simulink model "BESS1_pu"  (R2020b)
settings: Solver=ode1  StartTime=0.0  StopTime=160  FixedStep=Ts  RelTol=1e-3
PostLoadFcn:
  | clc; clear all; close all;
  | 
  | % Modulo 10 - Controle Grid-Forming %
  | 
  | vs_ref = 400;
  | Vnom_rms = vs_ref;
  | Vnom_peak = sqrt(2/3)*Vnom_rms;
  | Pnom =29.75e3;
  | Sbase = Pnom;
  | Vdc = 1400;
  | wnom = 2*pi*60;
  | ron = 0.00088;
  | Ron = ron;
  | %%%% To pu %%%%
  | Vbase = Vnom_rms*sqrt(2);
  | V_LG = Vnom_rms/sqrt(3);
  | Ibase = (Pnom*sqrt(2))/(V_LG*3);
  | 
  | Irms = Pnom/(sqrt(3)*Vnom_rms);                     % Ig rms
  | Inom_peak = Irms*sqrt(2);                           % Ig pico
  | Zbase = Vnom_peak/Inom_peak;                        % Impedancia Base
  | Kconv = Zbase;                                      % Ganho conversor
  | 
  | %%%% LCL Filter Project %%%%
  | fsw = 105*60;%105*60;                                         % switching frequency
  | ripple = 0.05;                                       % current ripple
  | L1 = Vdc/(6*ripple*Inom_peak*fsw);                  % inductor L1
  | R1 = 0.005;                                        % L1 resistance
  | Cbase = 1/(wnom*Kconv);                             % base capacitance
  | Cf = 0.05*Cbase;                                    % filter capacitor
  | Cf = 400e-6;
  | 
  | 
  | % Capacitor DC
  | C_cc_proj = (Sbase/(2*pi*60*Vdc*Vdc*0.05));
  | 
  | % Controladores
  | tau_i = 0.0005;
  | kp_corrente = L1/tau_i
  | ki_corrente = (R1+ron)/tau_i
  | kp_current_pu = kp_corrente/Kconv;                  % Adaptando para pu
  | ki_current_pu = ki_corrente/Kconv;
  | decouple_pu = (wnom*L1+(R1+Ron))/Kconv;
  | 
  | %decouple_i = wnom*L1
  | decouple_v = wnom*Cf
  | decouple_v_pu = (wnom*Cf)*Kconv;
  | 
  | % Controlador CA
  | S_Load = sqrt((25e3)^2+(20e3)^2);
  | Ibase_Load = ((S_Load*sqrt(2))/(V_LG*3))
  | 
  | 
  | a1=2
  | kp_tensao = Cf/(a1*tau_i)
  | Tn = 4*tau_i;
  | ki_tensao = kp_tensao/Tn
  | 
  | % To pu
  | Ica_pu = Pnom/Vdc;
  | ... (+28 lines)
InitFcn:
  | clc; clear all; close all;
  | 
  | % Modulo 10 - Controle Grid-Forming %
  | 
  | vs_ref = 400;
  | Vnom_rms = vs_ref;
  | Vnom_peak = sqrt(2/3)*Vnom_rms;
  | Pnom =29.75e3;
  | Sbase = Pnom;
  | Vdc = 1400;
  | wnom = 2*pi*60;
  | ron = 0.00088;
  | Ron = ron;
  | %%%% To pu %%%%
  | Vbase = Vnom_rms*sqrt(2);
  | V_LG = Vnom_rms/sqrt(3);
  | Ibase = (Pnom*sqrt(2))/(V_LG*3);
  | 
  | Irms = Pnom/(sqrt(3)*Vnom_rms);                     % Ig rms
  | Inom_peak = Irms*sqrt(2);                           % Ig pico
  | Zbase = Vnom_peak/Inom_peak;                        % Impedancia Base
  | Kconv = Zbase;                                      % Ganho conversor
  | 
  | %%%% LCL Filter Project %%%%
  | fsw = 105*60;%105*60;                                         % switching frequency
  | ripple = 0.05;                                       % current ripple
  | L1 = Vdc/(6*ripple*Inom_peak*fsw);                  % inductor L1
  | R1 = 0.005;                                        % L1 resistance
  | Cbase = 1/(wnom*Kconv);                             % base capacitance
  | Cf = 0.05*Cbase;                                    % filter capacitor
  | Cf = 400e-6;
  | 
  | 
  | % Capacitor DC
  | C_cc_proj = (Sbase/(2*pi*60*Vdc*Vdc*0.05));
  | 
  | % Controladores
  | tau_i = 0.0005;
  | kp_corrente = L1/tau_i
  | ki_corrente = (R1+ron)/tau_i
  | kp_current_pu = kp_corrente/Kconv;                  % Adaptando para pu
  | ki_current_pu = ki_corrente/Kconv;
  | decouple_pu = (wnom*L1+(R1+Ron))/Kconv;
  | 
  | %decouple_i = wnom*L1
  | decouple_v = wnom*Cf
  | decouple_v_pu = (wnom*Cf)*Kconv;
  | 
  | % Controlador CA
  | S_Load = sqrt((25e3)^2+(20e3)^2);
  | Ibase_Load = ((S_Load*sqrt(2))/(V_LG*3))
  | 
  | 
  | a1=2
  | kp_tensao = Cf/(a1*tau_i)
  | Tn = 4*tau_i;
  | ki_tensao = kp_tensao/Tn
  | 
  | % To pu
  | Ica_pu = Pnom/Vdc;
  | ... (+28 lines)
StartFcn:
  | clc; clear all; close all;
  | 
  | % Modulo 10 - Controle Grid-Forming %
  | 
  | vs_ref = 400;
  | Vnom_rms = vs_ref;
  | Vnom_peak = sqrt(2/3)*Vnom_rms;
  | Pnom =29.75e3;
  | Sbase = Pnom;
  | Vdc = 1400;
  | wnom = 2*pi*60;
  | ron = 0.00088;
  | Ron = ron;
  | %%%% To pu %%%%
  | Vbase = Vnom_rms*sqrt(2);
  | V_LG = Vnom_rms/sqrt(3);
  | Ibase = (Pnom*sqrt(2))/(V_LG*3);
  | 
  | Irms = Pnom/(sqrt(3)*Vnom_rms);                     % Ig rms
  | Inom_peak = Irms*sqrt(2);                           % Ig pico
  | Zbase = Vnom_peak/Inom_peak;                        % Impedancia Base
  | Kconv = Zbase;                                      % Ganho conversor
  | 
  | %%%% LCL Filter Project %%%%
  | fsw = 105*60;%105*60;                                         % switching frequency
  | ripple = 0.05;                                       % current ripple
  | L1 = Vdc/(6*ripple*Inom_peak*fsw);                  % inductor L1
  | R1 = 0.005;                                        % L1 resistance
  | Cbase = 1/(wnom*Kconv);                             % base capacitance
  | Cf = 0.05*Cbase;                                    % filter capacitor
  | Cf = 400e-6;
  | 
  | 
  | % Capacitor DC
  | C_cc_proj = (Sbase/(2*pi*60*Vdc*Vdc*0.05));
  | 
  | % Controladores
  | tau_i = 0.0005;
  | kp_corrente = L1/tau_i
  | ki_corrente = (R1+ron)/tau_i
  | kp_current_pu = kp_corrente/Kconv;                  % Adaptando para pu
  | ki_current_pu = ki_corrente/Kconv;
  | decouple_pu = (wnom*L1+(R1+Ron))/Kconv;
  | 
  | %decouple_i = wnom*L1
  | decouple_v = wnom*Cf
  | decouple_v_pu = (wnom*Cf)*Kconv;
  | 
  | % Controlador CA
  | S_Load = sqrt((25e3)^2+(20e3)^2);
  | Ibase_Load = ((S_Load*sqrt(2))/(V_LG*3))
  | 
  | 
  | a1=2
  | kp_tensao = Cf/(a1*tau_i)
  | Tn = 4*tau_i;
  | ki_tensao = kp_tensao/Tn
  | 
  | % To pu
  | Ica_pu = Pnom/Vdc;
  | ... (+28 lines)
undefined symbols (not defined in the file): DiscIntNeverNeededParam, I, Ion, Left, Lithium, ph, type, V
libraries: powerlib x18, powerlib_meascontrol x16, rtlab x6, artemis x2, eePowerMeasurement x2, rteventslib x2, ssn_inverter_model x1, electricdrivelib x1
(part 2 of 2)

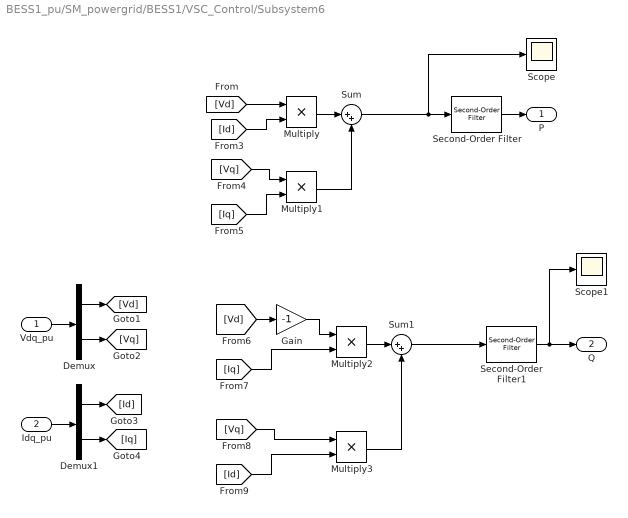
== system BESS1_pu/SM_powergrid/BESS1/VSC_Control/Subsystem6 ==
  Vdq_pu : Inport
  Idq_pu : Inport  Port=2
  Demux : Demux  Outputs=2
  Demux1 : Demux  Outputs=2
  Gain : Gain  Gain=-1
  Multiply{,1..3} (4 alike) : Product
  Scope : Scope
  Scope1 : Scope
  Second-Order Filter : powerlib_meascontrol/Filters/Second-Order Filter  FilterType=Lowpass  Fo=500  Zeta=1  Ts=Ts  Initialize=off  Vac_Init="[0,  0,  60]"  Vdc_Init=0  PlotResponse=off  FreqRange=[0, 500, 1]
      settings: SourceProductBaseCode=PS
  Second-Order Filter1 : powerlib_meascontrol/Filters/Second-Order Filter  FilterType=Lowpass  Fo=500  Zeta=1  Ts=Ts  Initialize=off  Vac_Init="[0,  0,  60]"  Vdc_Init=0  PlotResponse=off  FreqRange=[0, 500, 1]
      settings: SourceProductBaseCode=PS
  Sum : Sum  Inputs=|++
  Sum1 : Sum  Inputs=|++
  P : Outport  VectorParamsAs1DForOutWhenUnconnected=off
  Q : Outport  Port=2  VectorParamsAs1DForOutWhenUnconnected=off
  wires:
  Second-Order Filter1/1 -> Scope1/1, Q/1
  Second-Order Filter/1 -> P/1
  Sum1/1 -> Second-Order Filter1/1
  Demux/1 -> [Vd]
  Demux/2 -> [Vq]
  Demux1/1 -> [Id]
  Demux1/2 -> [Iq]
  [Vd] -> Multiply/1
  [Id] -> Multiply/2
  [Iq] -> Multiply1/2
  [Vq] -> Multiply1/1
  Multiply/1 -> Sum/1
  Multiply1/1 -> Sum/2
  Sum/1 -> Scope/1, Second-Order Filter/1
  Multiply3/1 -> Sum1/2
  Multiply2/1 -> Sum1/1
  [Vq] -> Multiply3/1
  [Id] -> Multiply3/2
  [Iq] -> Multiply2/2
  [Vd] -> Gain/1
  Gain/1 -> Multiply2/1
  Vdq_pu/1 -> Demux/1
  Idq_pu/1 -> Demux1/1

== system BESS1_pu/SM_powergrid/BESS1/VSC_Control/Transition ==
  Pref : Inport
  ilhamento : Inport  Port=2
  Idqref_F : Inport  Port=3
  Constant : Constant  Commented=on  Value=-0.8
  Constant1 : Constant  Value=0.75
  Divide : Product  Inputs=*/
  Divide1 : Product  Inputs=*/
  Gain : Gain  Gain=1/Pnom
  Gain1 : Gain  Gain=-2/3
  Mux1 : Mux  Inputs=2
  Product : Product
  Q_ref : Constant  Value=-25e3
  Rate Limiter : RateLimiter  SampleTimeMode=inherited
  Rate Limiter1 : RateLimiter  RisingSlewLimit=2000  FallingSlewLimit=-2000  SampleTimeMode=inherited
  Switch : Switch  Criteria=u2 > Threshold
  Vd_ref : Constant
  Vd_ref1 : Constant  Value=400/sqrt(3/2)
  Idq_ref : Outport
  wires:
  Vd_ref/1 -> Divide/2
  Gain/1 -> Divide/1
  Pref/1 -> Gain/1
  ilhamento/1 -> Product/2, Switch/2
  Switch/1 -> Idq_ref/1
  Idqref_F/1 -> Switch/3
  Q_ref/1 -> Gain1/1
  Gain1/1 -> Divide1/1
  Vd_ref1/1 -> Divide1/2
  Divide1/1 -> Rate Limiter1/1
  Constant1/1 -> Mux1/2
  Divide/1 -> Mux1/1
  Rate Limiter/1 -> Switch/1
  Mux1/1 -> Product/1
  Product/1 -> Rate Limiter/1

== system BESS1_pu/SM_powergrid/BESS1/VSC_Control/Uabc_ref Generation  ==
  note: Uabc_ref Generation
  wt : Inport
  m_dq : Inport  Port=2
  Constant5 : Constant  Value=0
  Mux : Mux  Inputs=2
  Scope : Scope
  dq0 to abc : powerlib_meascontrol/Transformations/dq0 to abc  Alignment=90 degrees behind phase A axis
  Uabc_ref : Outport  VectorParamsAs1DForOutWhenUnconnected=off
  wires:
  m_dq/1 -> Mux/1, Scope/1
  dq0 to abc/1 -> Uabc_ref/1
  wt/1 -> dq0 to abc/2
  Constant5/1 -> Mux/2
  Mux/1 -> dq0 to abc/1

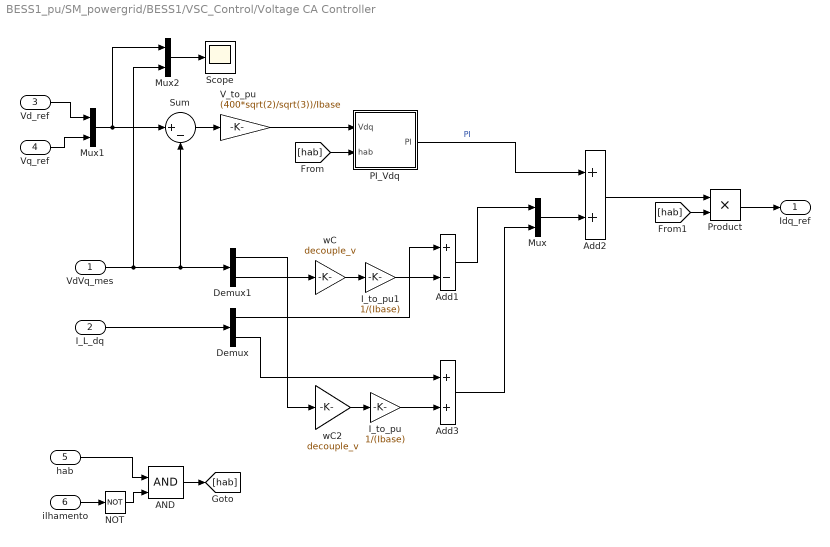
== system BESS1_pu/SM_powergrid/BESS1/VSC_Control/Voltage CA Controller ==
  VdVq_mes : Inport  PortDimensions=2
  I_L_dq : Inport  Port=2
  Vd_ref : Inport  Port=3  PortDimensions=1
  Vq_ref : Inport  Port=4
  hab : Inport  Port=5
  ilhamento : Inport  Port=6
  AND : Logic  IconShape=distinctive  AllPortsSameDT=off  OutDataTypeStr=boolean
  Add1 : Sum  Inputs=+-
  Add2 : Sum
  Add3 : Sum
  Demux : Demux  Outputs=2
  Demux1 : Demux  Outputs=2
  I_to_pu : Gain  Gain=1/(Ibase)  SaturateOnIntegerOverflow=on  OutDataTypeStr=Inherit: Same as input  ParamDataTypeStr=Inherit: Same as input
  I_to_pu1 : Gain  Gain=1/(Ibase)  SaturateOnIntegerOverflow=on  OutDataTypeStr=Inherit: Same as input  ParamDataTypeStr=Inherit: Same as input
  Mux : Mux  Inputs=2
  Mux1 : Mux  Inputs=2
  Mux2 : Mux  Inputs=2
  NOT : Logic  Operator=NOT  IconShape=distinctive  AllPortsSameDT=off  OutDataTypeStr=boolean
  PI_Vdq : Subsystem
  Product : Product
  Scope : Scope
  Sum : Sum  Inputs=|+-
  V_to_pu : Gain  Gain=(400*sqrt(2)/sqrt(3))/Ibase  SaturateOnIntegerOverflow=on  OutDataTypeStr=Inherit: Same as input  ParamDataTypeStr=Inherit: Same as input
  wC : Gain  Gain=decouple_v  SaturateOnIntegerOverflow=on  OutDataTypeStr=Inherit: Same as input  ParamDataTypeStr=Inherit: Same as input
  wC2 : Gain  Gain=decouple_v  SaturateOnIntegerOverflow=on  OutDataTypeStr=Inherit: Same as input  ParamDataTypeStr=Inherit: Same as input
  Idq_ref : Outport  SampleTime=Ts  InitialOutput=0  VectorParamsAs1DForOutWhenUnconnected=off
  wires:
  AND/1 -> [hab]
  hab/1 -> AND/1
  NOT/1 -> AND/2
  ilhamento/1 -> NOT/1
  [hab] -> PI_Vdq/2(hab)
  [hab] -> Product/2
  Product/1 -> Idq_ref/1
  Add2/1 -> Product/1
  Mux2/1 -> Scope/1
  VdVq_mes/1 -> Sum/2, Demux1/1, Mux2/2
  I_L_dq/1 -> Demux/1
  PI_Vdq/1(PI) -> Add2/1  "PI"
  Demux1/1 -> wC2/1
  wC/1 -> I_to_pu1/1
  Demux1/2 -> wC/1
  wC2/1 -> I_to_pu/1
  Mux/1 -> Add2/2
  Demux/1 -> Add1/1
  Demux/2 -> Add3/1
  Add1/1 -> Mux/1
  Add3/1 -> Mux/2
  Sum/1 -> V_to_pu/1
  V_to_pu/1 -> PI_Vdq/1(Vdq)
  I_to_pu/1 -> Add3/2
  I_to_pu1/1 -> Add1/2
  Mux1/1 -> Mux2/1, Sum/1
  Vd_ref/1 -> Mux1/1
  Vq_ref/1 -> Mux1/2

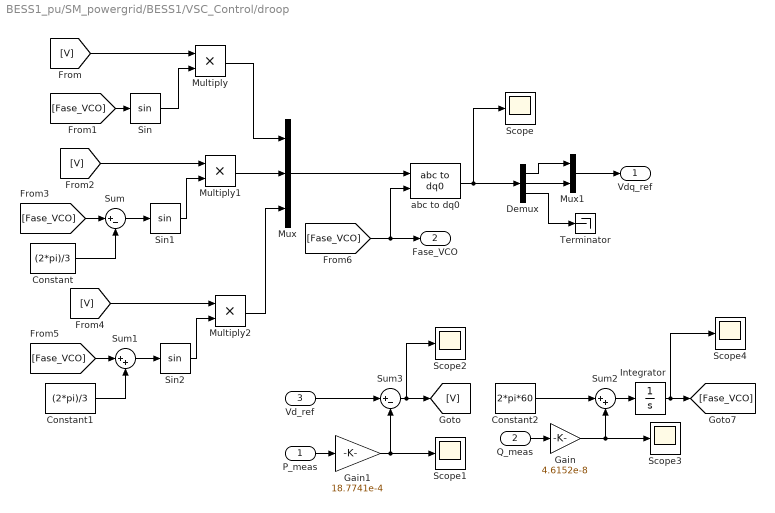
== system BESS1_pu/SM_powergrid/BESS1/VSC_Control/droop ==
  P_meas : Inport
  Q_meas : Inport  Port=2
  Vd_ref : Inport  Port=3
  Constant : Constant  Value=(2*pi)/3
  Constant1 : Constant  Value=(2*pi)/3
  Constant2 : Constant  Value=2*pi*60
  Demux : Demux  Outputs=3
  Gain : Gain  Gain=4.6152e-8
  Gain1 : Gain  Gain=18.7741e-4
  Integrator : Integrator  WrapState=on  WrappedStateUpperValue=2*pi  WrappedStateLowerValue=0
  Multiply : Product
  Multiply1 : Product
  Multiply2 : Product
  Mux : Mux  Inputs=3
  Mux1 : Mux  Inputs=2
  Scope{,1..4} (5 alike) : Scope
  Sin : Trigonometry
  Sin1 : Trigonometry
  Sin2 : Trigonometry
  Sum : Sum  Inputs=|+-
  Sum1 : Sum  Inputs=|++
  Sum2 : Sum  Inputs=|++
  Sum3 : Sum  Inputs=|+-
  Terminator : Terminator
  abc to dq0 : powerlib_meascontrol/Transformations/abc to dq0  Alignment=90 degrees behind phase A axis
  "Vdq_ref " : Outport  VectorParamsAs1DForOutWhenUnconnected=off
  "Fase_VCO " : Outport  Port=2  VectorParamsAs1DForOutWhenUnconnected=off
  wires:
  Q_meas/1 -> Gain/1
  P_meas/1 -> Gain1/1
  Gain1/1 -> Scope1/1, Sum3/2
  Gain/1 -> Scope3/1, Sum2/2
  Constant2/1 -> Sum2/1
  Vd_ref/1 -> Sum3/1
  Demux/3 -> Terminator/1
  abc to dq0/1 -> Demux/1, Scope/1
  [Fase_VCO] -> abc to dq0/2, "Fase_VCO "/1
  Mux/1 -> abc to dq0/1
  Multiply2/1 -> Mux/3
  Multiply1/1 -> Mux/2
  Multiply/1 -> Mux/1
  Sin2/1 -> Multiply2/2
  [V] -> Multiply2/1
  [Fase_VCO] -> Sum1/1
  Sum1/1 -> Sin2/1
  Constant1/1 -> Sum1/2
  Constant/1 -> Sum/2
  Sum/1 -> Sin1/1
  [Fase_VCO] -> Sum/1
  [V] -> Multiply1/1
  Sin1/1 -> Multiply1/2
  Sin/1 -> Multiply/2
  [V] -> Multiply/1
  [Fase_VCO] -> Sin/1
  Sum3/1 -> Scope2/1, [V]
  Sum2/1 -> Integrator/1
  Integrator/1 -> Scope4/1, [Fase_VCO]
  Demux/1 -> Mux1/1
  Demux/2 -> Mux1/2
  Mux1/1 -> "Vdq_ref "/1

== system BESS1_pu/SM_powergrid/BESS1/VSC_Control/Current Controller/PI_Idq ==
  Vdq : Inport
  hab : Inport  Port=2
  Discrete-Time Integrator : DiscreteIntegrator  SampleTime=-1  ICPrevOutput=DiscIntNeverNeededParam  ICPrevScaledInput=DiscIntNeverNeededParam
  Gain1 : Gain  Gain=kp_current_pu
  Gain2 : Gain  Gain=ki_current_pu
  Product : Product
  Sum1 : Sum
  PI : Outport
  wires:
  hab/1 -> Product/2
  Vdq/1 -> Product/1
  Discrete-Time Integrator/1 -> Sum1/2
  Sum1/1 -> PI/1
  Gain1/1 -> Sum1/1
  Product/1 -> Gain2/1, Gain1/1
  Gain2/1 -> Discrete-Time Integrator/1

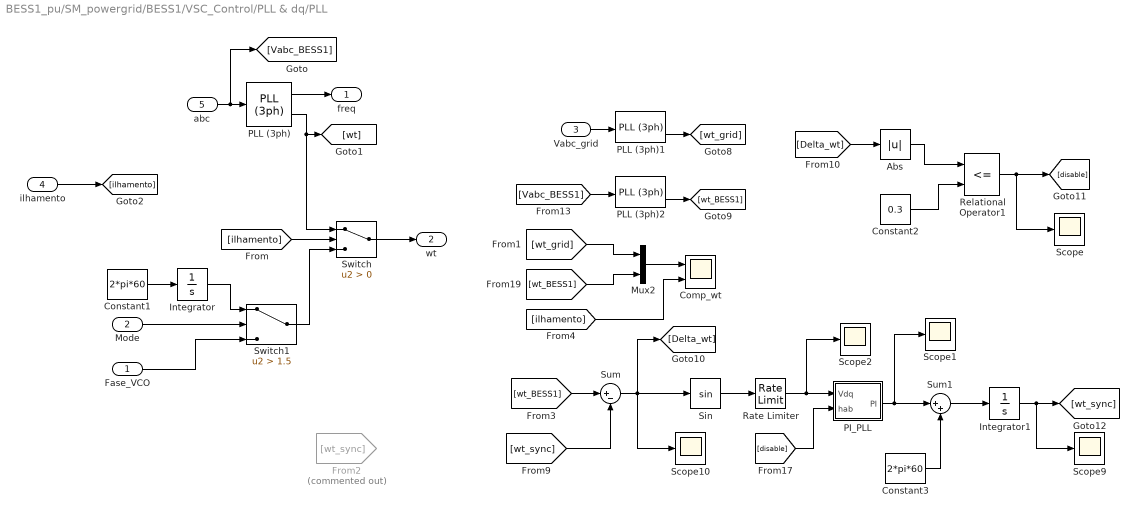
== system BESS1_pu/SM_powergrid/BESS1/VSC_Control/PLL & dq/PLL ==
  "Fase_VCO " : Inport
  Mode : Inport  Port=2
  Vabc_grid : Inport  Port=3
  ilhamento : Inport  Port=4
  abc : Inport  Port=5
  Abs : Abs
  Comp_wt : Scope  NumInputPorts=2
  Constant1 : Constant  Value=2*pi*60
  Constant2 : Constant  Value=0.3
  Constant3 : Constant  Value=2*pi*60
  From2 : From  Commented=on  GotoTag=wt_sync
  Integrator : Integrator  WrapState=on  WrappedStateUpperValue=2*pi  WrappedStateLowerValue=0
  Integrator1 : Integrator  WrapState=on  WrappedStateUpperValue=2*pi  WrappedStateLowerValue=0
  Mux2 : Mux  Inputs=2
  PI_PLL : Subsystem
  PLL (3ph) : powerlib_meascontrol/PLL/PLL (3ph)  Fmin=45  Par_Init="[-0.57  60]"  ParK=[180, 3200, 1]  TcD=Ts_Control  MaxRateChangeFreq=12  FilterCutOffFreq=25  Ts=Ts_Control  AGC=on
  PLL (3ph)1 : powerlib_meascontrol/PLL/PLL (3ph)  Fmin=55  Par_Init=[0, 60]  ParK=[180, 3200, 1]  TcD=1e-4  MaxRateChangeFreq=12  FilterCutOffFreq=25  Ts=0  AGC=on
  PLL (3ph)2 : powerlib_meascontrol/PLL/PLL (3ph)  Fmin=55  Par_Init=[0, 60]  ParK=[180, 3200, 1]  TcD=1e-4  MaxRateChangeFreq=12  FilterCutOffFreq=25  Ts=0  AGC=on
  Rate Limiter : RateLimiter  RisingSlewLimit=10  FallingSlewLimit=-10  SampleTimeMode=inherited
  Relational Operator1 : RelationalOperator  Operator=<=  OutDataTypeStr=boolean  RndMeth=Simplest
  Scope{,1..2,9..10} (5 alike) : Scope
  Sin : Trigonometry
  Sum : Sum  Inputs=|+-
  Sum1 : Sum  Inputs=|++
  Switch : Switch  Criteria=u2 > Threshold
  Switch1 : Switch  Criteria=u2 > Threshold  Threshold=1.5
  freq : Outport
  wt : Outport  Port=2
  wires:
  Switch/1 -> wt/1
  PLL (3ph)/2 -> [wt], Switch/1
  PI_PLL/1(PI) -> Sum1/1, Scope1/1
  "Fase_VCO "/1 -> Switch1/3
  Switch1/1 -> Switch/3
  Mode/1 -> Switch1/2
  Integrator/1 -> Switch1/1
  Constant1/1 -> Integrator/1
  [Vabc_BESS1] -> PLL (3ph)2/1
  [wt_BESS1] -> Mux2/2
  [wt_sync] -> Sum/2
  Abs/1 -> Relational Operator1/1
  Sum/1 -> Sin/1, [Delta_wt], Scope10/1
  Relational Operator1/1 -> [disable], Scope/1
  Constant3/1 -> Sum1/2
  Rate Limiter/1 -> PI_PLL/1(Vdq), Scope2/1
  [Delta_wt] -> Abs/1
  Constant2/1 -> Relational Operator1/2
  [wt_grid] -> Mux2/1
  Mux2/1 -> Comp_wt/1
  [disable] -> PI_PLL/2(hab)
  [wt_BESS1] -> Sum/1
  PLL (3ph)2/2 -> [wt_BESS1]
  Sin/1 -> Rate Limiter/1
  Sum1/1 -> Integrator1/1
  Integrator1/1 -> [wt_sync], Scope9/1
  PLL (3ph)1/2 -> [wt_grid]
  Vabc_grid/1 -> PLL (3ph)1/1
  abc/1 -> PLL (3ph)/1, [Vabc_BESS1]
  PLL (3ph)/1 -> freq/1
  ilhamento/1 -> [ilhamento]
  [ilhamento] -> Switch/2
  [ilhamento] -> Comp_wt/2

== system BESS1_pu/SM_powergrid/BESS1/VSC_Control/PLL & dq/filtro2 ==
  dq : Inport
  Demux : Demux  Outputs=2
  Mux1 : Mux  Inputs=2
  Transfer Fcn1 : TransferFcn  Denominator=[2.53e-4 1]
  Transfer Fcn2 : TransferFcn  Denominator=[2.53e-4 1]
  dq_filter : Outport
  wires:
  Mux1/1 -> dq_filter/1
  dq/1 -> Demux/1
  Transfer Fcn1/1 -> Mux1/1
  Demux/2 -> Transfer Fcn2/1
  Demux/1 -> Transfer Fcn1/1
  Transfer Fcn2/1 -> Mux1/2

== system BESS1_pu/SM_powergrid/BESS1/VSC_Control/Voltage CA Controller/PI_Vdq ==
  Vdq : Inport
  hab : Inport  Port=2
  Discrete-Time Integrator : DiscreteIntegrator  SampleTime=-1  ICPrevOutput=DiscIntNeverNeededParam  ICPrevScaledInput=DiscIntNeverNeededParam
  Gain1 : Gain  Gain=kp_tensao
  Gain2 : Gain  Gain=ki_tensao
  Product : Product
  Sum1 : Sum
  PI : Outport
  wires:
  hab/1 -> Product/2
  Vdq/1 -> Product/1
  Discrete-Time Integrator/1 -> Sum1/2
  Sum1/1 -> PI/1
  Gain1/1 -> Sum1/1
  Product/1 -> Gain2/1, Gain1/1
  Gain2/1 -> Discrete-Time Integrator/1

== system BESS1_pu/SM_powergrid/BESS1/VSC_Control/PLL & dq/PLL/PI_PLL ==
  Vdq : Inport
  hab : Inport  Port=2
  Discrete-Time Integrator : DiscreteIntegrator  SampleTime=-1  ICPrevOutput=DiscIntNeverNeededParam  ICPrevScaledInput=DiscIntNeverNeededParam
  Gain1 : Gain  Gain=400
  Gain2 : Gain  Gain=40
  Product : Product
  Product1 : Product
  Sum1 : Sum
  PI : Outport
  wires:
  Product1/1 -> PI/1
  Sum1/1 -> Product1/1
  hab/1 -> Product/2, Product1/2
  Vdq/1 -> Product/1
  Discrete-Time Integrator/1 -> Sum1/2
  Gain1/1 -> Sum1/1
  Product/1 -> Gain2/1, Gain1/1
  Gain2/1 -> Discrete-Time Integrator/1
